simulink model "Pnt"  (R2020b)
settings: configuration reference "gen_config" (kept outside this file)
undefined symbols (not defined in the file): Pnt_capBat_C, Pnt_facSocInit_C, Pnt_resBatInner_C
settings Model: DataDictionary=Hybrid_vehicle_update.sldd  SimulationMode=accelerator  Creator=Georg  LastModifiedBy=jy
settings ConfigSetRef: SourceName=gen_config

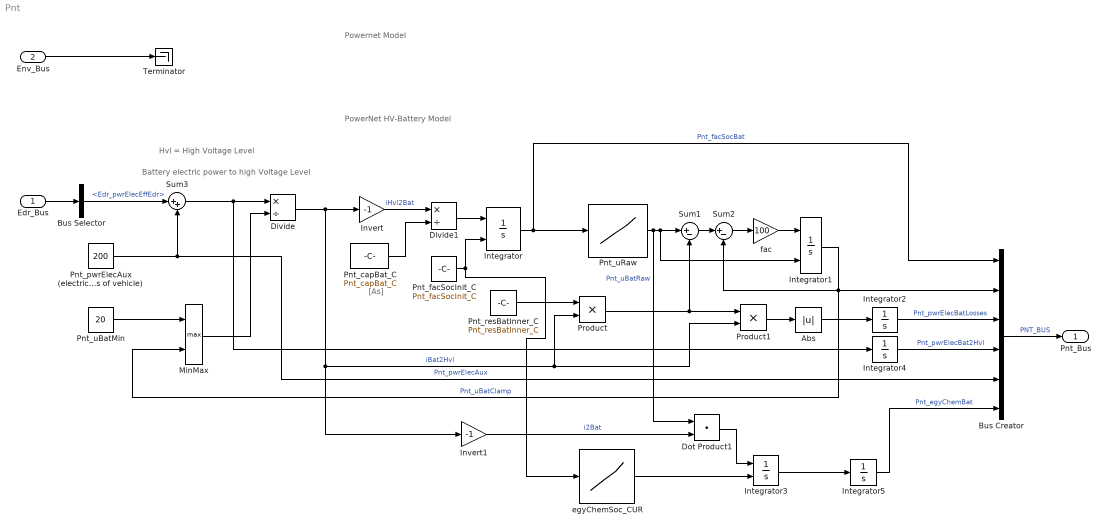
== system Pnt ==
  note: Hvl = High Voltage Level
  note: Battery electric power to high Voltage Level
  note: PowerNet HV-Battery Model
  note: [As]
  note: Powernet Model
  Edr_Bus : Inport  OutDataTypeStr=Bus: EDR_BUS
  Env_Bus : Inport  Port=2  OutDataTypeStr=Bus: ENV_BUS
  Abs : Abs
  Bus Creator : BusCreator  Inputs=6  OutDataTypeStr=Bus: PNT_BUS  NonVirtualBus=on
  Bus Selector : BusSelector  OutputSignals=Edr_pwrElecEffEdr
  Divide : Product  Inputs=*/
  Divide1 : Product  Inputs=*/
  Dot Product1 : DotProduct  InputSameDT=on  OutDataTypeStr=Inherit: Inherit via internal rule
  Integrator : Integrator  InitialConditionSource=external  InitialCondition=0.8  LimitOutput=on  UpperSaturationLimit=1  LowerSaturationLimit=0
  Integrator1 : Integrator  InitialConditionSource=external  InitialCondition=0.8
  Integrator2 : Integrator
  Integrator3 : Integrator  InitialConditionSource=external
  Integrator4 : Integrator
  Integrator5 : Integrator
  Invert : Gain  Gain=-1
  Invert1 : Gain  Gain=-1
  MinMax : MinMax  Function=max  Inputs=2
  Pnt_capBat_C : Constant  Value=Pnt_capBat_C
  Pnt_facSocInit_C : Constant  Value=Pnt_facSocInit_C
  Pnt_pwrElecAux (electric auxilliaries of vehicle) : Constant  Value=200
  Pnt_resBatInner_C : Constant  Value=Pnt_resBatInner_C
  Pnt_uBatMin : Constant  Value=20
  Pnt_uRaw : Lookup  InputValues="[0, 0.1 0.2  0.5  0.8  1]"  Table="[50 250  290   350  385  400]"  LookUpMeth=Interpolation-Use End Values
  Product : Product  RndMeth=Zero
  Product1 : Product  RndMeth=Zero
  Sum1 : Sum  Inputs=|+-
  Sum2 : Sum  Inputs=|+-
  Sum3 : Sum  Inputs=|++
  Terminator : Terminator
  egyChemSoc_CUR : Lookup_n-D  NumberOfTableDimensions=1  BreakpointsForDimension1=[0 0.05 0.1 0.2 0.3 0.4 0.5 0.6 0.7 0.8 0.9 1]  Table=[0 2.751 8.13 22.73 38.87 56.19 74.6 93.75 113.6 134.2 155.1 176.5 ]*10^5  InternalRulePriority=Speed  RndMeth=Simplest  InputSameDT=on
  fac : Gain  Gain=100
  Pnt_Bus : Outport  OutDataTypeStr=Bus: PNT_BUS  VectorParamsAs1DForOutWhenUnconnected=off
  wires:
  Sum3/1 -> Integrator4/1, Divide/1
  Integrator5/1 -> Bus Creator/6  "Pnt_egyChemBat"
  Pnt_pwrElecAux (electric auxilliaries of vehicle)/1 -> Bus Creator/5, Sum3/2  "Pnt_pwrElecAux"
  Product1/1 -> Abs/1
  Dot Product1/1 -> Integrator3/1
  Env_Bus/1 -> Terminator/1
  Invert1/1 -> Dot Product1/2  "i2Bat"
  Pnt_uRaw/1 -> Dot Product1/1, Integrator1/2, Sum1/1  "Pnt_uBatRaw"
  Integrator4/1 -> Bus Creator/4  "Pnt_pwrElecBat2Hvl"
  Integrator1/1 -> Sum2/2, Bus Creator/2, MinMax/2  "Pnt_uBatClamp"
  Pnt_capBat_C/1 -> Divide1/2
  egyChemSoc_CUR/1 -> Integrator3/2
  Divide/1 -> Invert/1, Invert1/1, Product/2, Product1/2  "iBat2Hvl"
  Pnt_facSocInit_C/1 -> Integrator/2, egyChemSoc_CUR/1
  Pnt_uBatMin/1 -> MinMax/1
  fac/1 -> Integrator1/1
  Sum1/1 -> Sum2/1
  Sum2/1 -> fac/1
  Abs/1 -> Integrator2/1
  Divide1/1 -> Integrator/1
  MinMax/1 -> Divide/2
  Edr_Bus/1 -> Bus Selector/1
  Pnt_resBatInner_C/1 -> Product/1
  Invert/1 -> Divide1/1  "iHvl2Bat"
  Bus Creator/1 -> Pnt_Bus/1  "PNT_BUS"
  Bus Selector/1 -> Sum3/1  "<Edr_pwrElecEffEdr>"
  Integrator3/1 -> Integrator5/1
  Integrator2/1 -> Bus Creator/3  "Pnt_pwrElecBatLosses"
  Product/1 -> Sum1/2, Product1/1
  Integrator/1 -> Pnt_uRaw/1, Bus Creator/1  "Pnt_facSocBat"
